simulink model "exercicio_3_1_sim"  (R2018a)
settings: Solver=VariableStepAuto  StartTime=0.0  StopTime=20.0  RelTol=1e-3
values from neighbouring files (symbols this model uses):
  D_amp = 1    [exercicio_3_1.m]    (also in exercicio_3_2.m)
  D_time = 50    [exercicio_3_1.m]    (also in exercicio_3_2.m = 10)
  den = [1 7 6 0]    [exercicio_1_3.m]    (also in exercicio_3_1.m = [1 2.5 1 0]; exercicio_3_2.m = [1 3.74 0]; simplifica_funcao.m = [1 7 16 30])
  Kd = Kp * Td    (= 2.35619449019)    [exercicio_3_1.m]    (also in exercicio_3_2.m = (p + 2*phi*wn - a1)/b0)
  Ki = Kp / Ti    (= 0.954929658551)    [exercicio_3_1.m]    (also in exercicio_3_2.m = (p*wn^2)/b0)
  Kp = 0.6 * Kp_crit    (= 3)    [exercicio_3_1.m]    (also in exercicio_3_2.m = (2*phi*wn*p + wn^2 - a0)/b0)
  num = [2 6]    [exercicio_1_3.m]    (also in exercicio_3_1.m = [0.5]; exercicio_3_2.m = [2.05])
  R_amp = 1    [exercicio_3_1.m]    (also in exercicio_3_2.m)
  R_time = 1    [exercicio_3_1.m]    (also in exercicio_3_2.m)
libraries: simulink x1
settings Model: Creator=Eduardo Rodrigues  LastModifiedBy=Eduardo Rodrigues

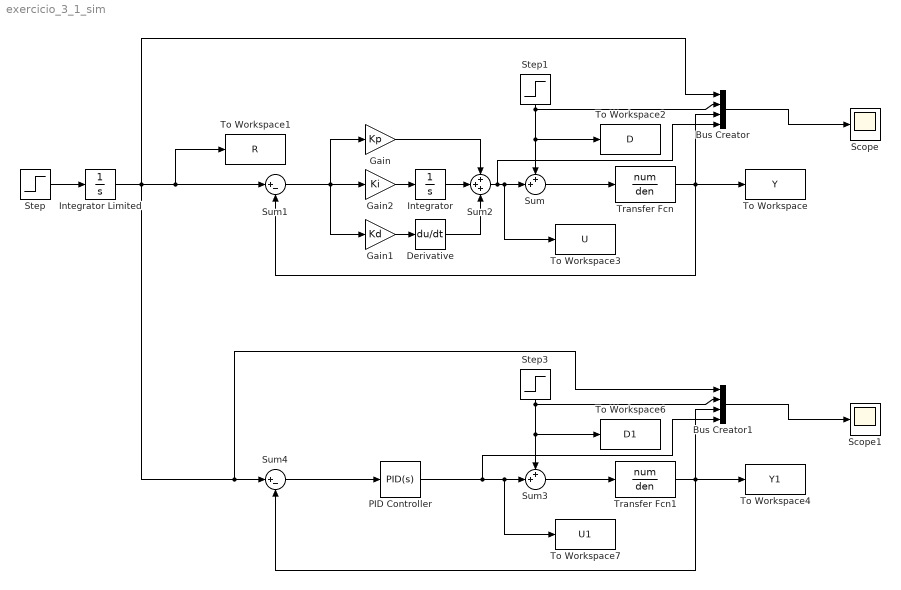
== system exercicio_3_1_sim ==
  Bus Creator : BusCreator  Inputs=4
  Bus Creator1 : BusCreator  Inputs=4
  Derivative : Derivative  CoefficientInTFapproximation=0
  Gain : Gain  Gain=Kp
  Gain1 : Gain  Gain=Kd
  Gain2 : Gain  Gain=Ki
  Integrator : Integrator
  Integrator Limited : Integrator  LimitOutput=on  UpperSaturationLimit=R_amp  LowerSaturationLimit=0
  PID Controller : simulink/Continuous/PID Controller  Controller=PID  TimeDomain=Continuous-time  SampleTime=-1  IntegratorMethod=Forward Euler  FilterMethod=Forward Euler  Form=Parallel  UseFilter=on  ControllerParametersSource=internal  P=Kp  I=Ki  D=Kd  N=100  InitialConditionSource=internal  InitialConditionForIntegrator=0  InitialConditionForFilter=0  ExternalReset=none  LimitOutput=off  UpperSaturationLimit=inf  LowerSaturationLimit=-inf  LinearizeAsGain=on  AntiWindupMode=none  Kb=1  TrackingMode=off  Kt=1  PParamMin=[]  PParamMax=[]  IParamMin=[]  IParamMax=[]  DParamMin=[]  DParamMax=[]  NParamMin=[]  NParamMax=[]  KbParamMin=[]  KbParamMax=[]  KtParamMin=[]  KtParamMax=[]  POutMin=[]  POutMax=[]  IOutMin=[]  IOutMax=[]  DOutMin=[]  DOutMax=[]  NOutMin=[]  NOutMax=[]  KbOutMin=[]  KbOutMax=[]  KtOutMin=[]  KtOutMax=[]  IntegratorOutMin=[]  IntegratorOutMax=[]  FilterOutMin=[]  FilterOutMax=[]  SumOutMin=[]  SumOutMax=[]  SumI1OutMin=[]  SumI1OutMax=[]  SumI2OutMin=[]  SumI2OutMax=[]  SumI3OutMin=[]  SumI3OutMax=[]  SumDOutMin=[]  SumDOutMax=[]  SaturationOutMin=[]  SaturationOutMax=[]  IntegratorContinuousStateAttributes=''  IntegratorStateMustResolveToSignalObject=off  IntegratorRTWStateStorageClass=Auto  FilterContinuousStateAttributes=''  FilterStateMustResolveToSignalObject=off  FilterRTWStateStorageClass=Auto  DifferentiatorICPrevScaledInput=0  DifferentiatorOutMin=[]  DifferentiatorOutMax=[]  FilterDiffOutCoefMin=[]  FilterDiffOutCoefMax=[]  SumDenOutMin=[]  SumDenOutMax=[]  SumNumOutMin=[]  SumNumOutMax=[]  ReciprocalOutMin=[]  ReciprocalOutMax=[]  DivideOutMin=[]  DivideOutMax=[]  TunerSelectOption=Transfer Function Based (PID Tuner App)
  Scope : Scope
  Scope1 : Scope
  Step : Step  Time=R_time  After=R_amp  SampleTime=0
  Step1 : Step  Time=D_time  After=D_amp  SampleTime=0
  Step3 : Step  Time=D_time  After=D_amp  SampleTime=0
  Sum : Sum  Inputs=++|
  Sum1 : Sum  Inputs=|+-
  Sum2 : Sum  Inputs=+++
  Sum3 : Sum  Inputs=++|
  Sum4 : Sum  Inputs=|+-
  To Workspace : ToWorkspace  VariableName=Y  SaveFormat=Structure With Time  SampleTime=-1
  To Workspace1 : ToWorkspace  VariableName=R  SaveFormat=Structure With Time  SampleTime=-1
  To Workspace2 : ToWorkspace  VariableName=D  SaveFormat=Structure With Time  SampleTime=-1
  To Workspace3 : ToWorkspace  VariableName=U  SaveFormat=Timeseries  SampleTime=-1
  To Workspace4 : ToWorkspace  VariableName=Y1  SaveFormat=Structure With Time  SampleTime=-1
  To Workspace6 : ToWorkspace  VariableName=D1  SaveFormat=Structure With Time  SampleTime=-1
  To Workspace7 : ToWorkspace  VariableName=U1  SaveFormat=Timeseries  SampleTime=-1
  Transfer Fcn : TransferFcn  Numerator=num  Denominator=den
  Transfer Fcn1 : TransferFcn  Numerator=num  Denominator=den
  wires:
  Bus Creator/1 -> Scope/1
  Transfer Fcn/1 -> To Workspace/1, Bus Creator/3, Sum1/2
  Sum1/1 -> Gain2/1, Gain1/1, Gain/1
  Step1/1 -> To Workspace2/1, Sum/1, Bus Creator/2
  Sum/1 -> Transfer Fcn/1
  Sum2/1 -> Bus Creator/4, To Workspace3/1, Sum/2
  Gain/1 -> Sum2/1
  Gain2/1 -> Integrator/1
  Integrator/1 -> Sum2/2
  Gain1/1 -> Derivative/1
  Derivative/1 -> Sum2/3
  PID Controller/1 -> Bus Creator1/4, To Workspace7/1, Sum3/2
  Sum3/1 -> Transfer Fcn1/1
  Transfer Fcn1/1 -> To Workspace4/1, Bus Creator1/3, Sum4/2
  Step3/1 -> To Workspace6/1, Sum3/1, Bus Creator1/2
  Bus Creator1/1 -> Scope1/1
  Sum4/1 -> PID Controller/1
  Step/1 -> Integrator Limited/1
  Integrator Limited/1 -> Bus Creator1/1, Sum4/1, To Workspace1/1, Sum1/1, Bus Creator/1
